simulink model "PTC_MBDS_DateTimeDisassemble_Sample"  (R2013a)
settings: Solver=FixedStepDiscrete  StartTime=0.0  StopTime=Inf  FixedStep=0.01  RelTol=1e-3
libraries: PTC_MBDS_LIB x2, simulink_extras x1
settings Model: Creator=Jordan.Mosher  LastModifiedBy=sundeep.tuteja

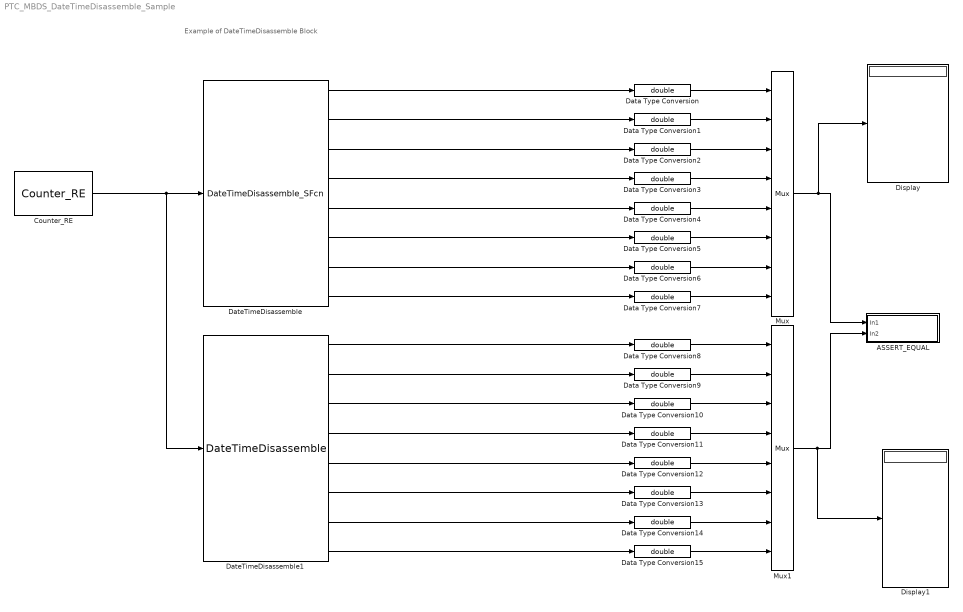
== system PTC_MBDS_DateTimeDisassemble_Sample ==
  note: Example of DateTimeDisassemble Block
  ASSERT_EQUAL : Subsystem
  Counter_RE : PTC_MBDS_LIB/MBDS Standard Library/Extended Operations/Counter & Timer/Counter_RE  E_Enabled=off  R_Enabled=off  IV_Enabled=off  IV=0  OutDataTypeStr=uint32  PTC_MBDS_BlockVersion=5.40  PTC_BlockType=PTC_MBDS_Counter_RE
      settings: AttributesFormatString=IV = %<IV>
  Data Type Conversion{,1..15} (16 alike) : DataTypeConversion  OutDataTypeStr=double  SaturateOnIntegerOverflow=on
  DateTimeDisassemble : S-Function  InitFcn=|  FunctionName=DateTimeDisassemble_SFcn  Parameters=boolean(ENO_Enabled)  EnableBusSupport=off  mask(DateTimeDisassemble){MBDS_LibraryBlock=on, ENO_Enabled=on, MBDS_BlockVersion=05.41}
      | if(exist('MBDS_BlockCallback', 'file'))
      |    MBDS_BlockCallback('Update', gcb);  
      | end
      mask prompts: MBDS_LibraryBlock "MBDS Library Block"; ENO_Enabled "Show ENO port"; MBDS_BlockVersion "Block version:"
      mask help: Disassembles a date_time signal into its date time components, i.e. year, month, day, hour, minute, second. Additionally the day of week number is output. If the input signal is invalid the ENO output is false.
      mask init:
      | MBDS_BlockCallback('Copy', gcb);                                        
      | maskdisplay = 'disp(sprintf(''Date Time\nDisassemble''))';
      | maskdisplay = [maskdisplay 10 'port_label(''output'', 1, ''Year'')' 10];
      | maskdisplay = [maskdisplay 'port_label(''output'', 2, ''Month'')' 10];
      | maskdisplay = [maskdisplay 'port_label(''output'', 3, ''Day'')' 10];
      | maskdisplay = [maskdisplay 'port_label(''output'', 4, ''Hours'')' 10];
      | maskdisplay = [maskdisplay 'port_label(''output'', 5, ''Minutes'')' 10];
      | maskdisplay = [maskdisplay 'port_label(''output'', 6, ''Seconds'')' 10];
      | maskdisplay = [maskdisplay 'port_label(''output'', 7, ''Day of Week'')' 10];
      | if(ENO_Enabled)
      |     maskdisplay = [maskdisplay 'port_label(''output'', 8, ''ENO'')' 10];
      | end
      | maskdisplay = [maskdisplay 'port_label(''input'', 1, ''DT'')' 10];
      | set_param(gcbh, 'maskdisplay', maskdisplay)
      | UpdateBlockSize(gcb);
      mask Help: eval(['open([workdir(''RT_Dir:''),''\Host\Library\Blockset\Help\'',get_param(gcb,''MaskType''),''.html''])']);
      mask Display:
      | disp(sprintf('Date Time\nDisassemble'))
      | port_label('output', 1, 'Year')
      | port_label('output', 2, 'Month')
      | port_label('output', 3, 'Day')
      | port_label('output', 4, 'Hours')
      | port_label('output', 5, 'Minutes')
      | port_label('output', 6, 'Seconds')
      | port_label('output', 7, 'Day of Week')
      | port_label('output', 8, 'ENO')
      | port_label('input', 1, 'DT')
  DateTimeDisassemble1 : PTC_MBDS_LIB/MBDS Standard Library/Extended Operations/Date & Time Operations/Date & Time Conversions/DateTimeDisassemble  ENO_Enabled=on  PTC_MBDS_BlockVersion=5.40  PTC_BlockType=PTC_MBDS_DateTimeDisassemble
  Display : Display
  Display1 : Display
  Mux : Mux  Inputs=8
  Mux1 : Mux  Inputs=8
  wires:
  Counter_RE/1 -> DateTimeDisassemble1/1, DateTimeDisassemble/1
  DateTimeDisassemble/5 -> Data Type Conversion4/1
  DateTimeDisassemble/4 -> Data Type Conversion3/1
  DateTimeDisassemble/3 -> Data Type Conversion2/1
  DateTimeDisassemble/7 -> Data Type Conversion6/1
  DateTimeDisassemble/6 -> Data Type Conversion5/1
  DateTimeDisassemble/1 -> Data Type Conversion/1
  DateTimeDisassemble/8 -> Data Type Conversion7/1
  DateTimeDisassemble/2 -> Data Type Conversion1/1
  DateTimeDisassemble1/1 -> Data Type Conversion8/1
  DateTimeDisassemble1/2 -> Data Type Conversion9/1
  DateTimeDisassemble1/3 -> Data Type Conversion10/1
  DateTimeDisassemble1/4 -> Data Type Conversion11/1
  DateTimeDisassemble1/5 -> Data Type Conversion12/1
  DateTimeDisassemble1/6 -> Data Type Conversion13/1
  DateTimeDisassemble1/7 -> Data Type Conversion14/1
  DateTimeDisassemble1/8 -> Data Type Conversion15/1
  Data Type Conversion3/1 -> Mux/4
  Data Type Conversion4/1 -> Mux/5
  Data Type Conversion2/1 -> Mux/3
  Data Type Conversion5/1 -> Mux/6
  Data Type Conversion1/1 -> Mux/2
  Data Type Conversion6/1 -> Mux/7
  Data Type Conversion/1 -> Mux/1
  Data Type Conversion7/1 -> Mux/8
  Data Type Conversion15/1 -> Mux1/8
  Data Type Conversion14/1 -> Mux1/7
  Data Type Conversion13/1 -> Mux1/6
  Data Type Conversion12/1 -> Mux1/5
  Data Type Conversion11/1 -> Mux1/4
  Data Type Conversion10/1 -> Mux1/3
  Data Type Conversion9/1 -> Mux1/2
  Data Type Conversion8/1 -> Mux1/1
  Mux1/1 -> Display1/1, ASSERT_EQUAL/2(In2)
  Mux/1 -> Display/1, ASSERT_EQUAL/1(In1)

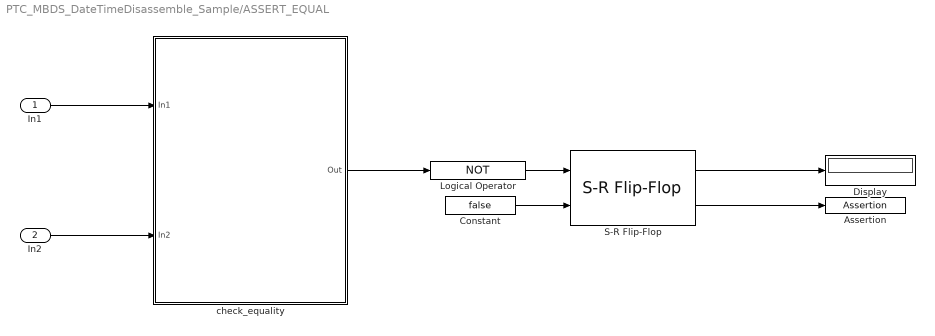
== system PTC_MBDS_DateTimeDisassemble_Sample/ASSERT_EQUAL ==
  In1 : Inport
  In2 : Inport  Port=2
  Assertion : Assertion
  Constant : Constant  Value=false
  Display : Display
  Logical Operator : Logic  Operator=NOT  AllPortsSameDT=off  OutDataTypeStr=boolean
  S-R Flip-Flop : simulink_extras/Flip Flops/S-R Flip-Flop  initial_condition=0
  check_equality : MATLAB Function  TreatAsAtomicUnit=on
  wires:
  S-R Flip-Flop/1 -> Display/1
  check_equality/1(Out) -> Logical Operator/1
  Constant/1 -> S-R Flip-Flop/2
  S-R Flip-Flop/2 -> Assertion/1
  In2/1 -> check_equality/2(In2)
  In1/1 -> check_equality/1(In1)
  Logical Operator/1 -> S-R Flip-Flop/1

== matlab function PTC_MBDS_DateTimeDisassemble_Sample/ASSERT_EQUAL/check_equality ==
  data: In1 input; Out output; In2 input
function Out = check_equality(In1, In2)
%#codegen

Out = isequaln(In1, In2);

end
